simulink model "data"  (R2022a)
settings: Solver=ode1  StartTime=0.0  StopTime=100  FixedStep=0.001  RelTol=1e-3
libraries: roblocks x4
settings Model: Creator=DELL  LastModifiedBy=qinyi
settings DebuggingCC: UnconnectedInputMsg=warning  UnconnectedOutputMsg=warning  UnconnectedLineMsg=warning
settings RTWCC: DLArmComputeVersion=19.05

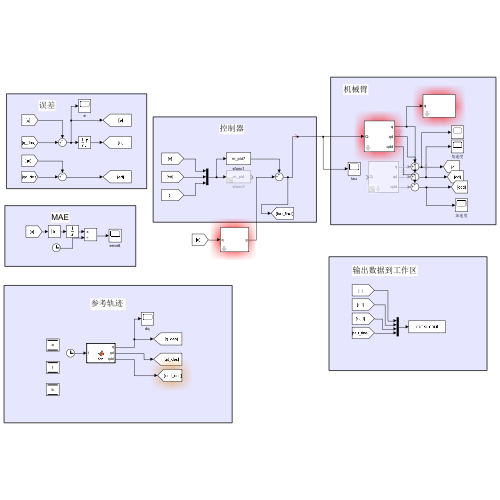
[thumbnail: Simulink's stored preview of the top-level diagram]
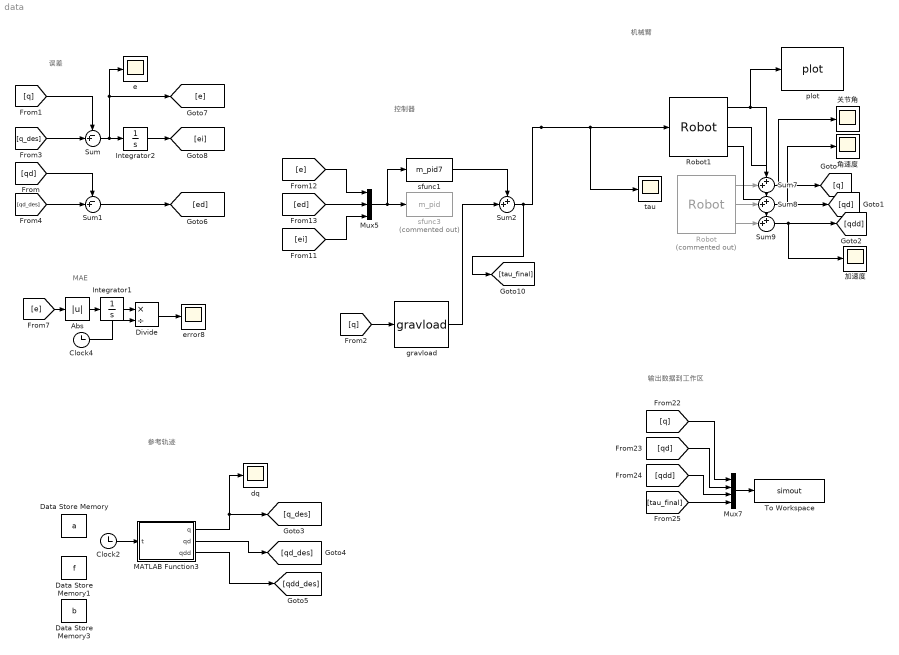
== system data ==
  note: MAE
  note: 机械臂
  note: 控制器
  note: 误差
  note: 参考轨迹
  note: 输出数据到工作区
  Abs : Abs  SaturateOnIntegerOverflow=off
  Clock2 : Clock
  Clock4 : Clock
  Data Store Memory : DataStoreMemory  DataStoreName=a  ReadBeforeWriteMsg=warning  WriteAfterWriteMsg=warning  WriteAfterReadMsg=warning  InitialValue=rand(10,7)  ShowAdditionalParam=off  OutDataTypeStr=double
  Data Store Memory1 : DataStoreMemory  DataStoreName=f  ReadBeforeWriteMsg=warning  WriteAfterWriteMsg=warning  WriteAfterReadMsg=warning  InitialValue=rand(10,7)  ShowAdditionalParam=off  OutDataTypeStr=double
  Data Store Memory3 : DataStoreMemory  DataStoreName=b  ReadBeforeWriteMsg=warning  WriteAfterWriteMsg=warning  WriteAfterReadMsg=warning  InitialValue=rand(10,7)  ShowAdditionalParam=off  OutDataTypeStr=double
  Divide : Product  Inputs=*/
  Integrator1 : Integrator
  Integrator2 : Integrator  LimitOutput=on  UpperSaturationLimit=0.01  LowerSaturationLimit=-0.01
  MATLAB Function3 : MATLAB Function  TreatAsAtomicUnit=on
  Mux5 : Mux  Inputs=3
  Mux7 : Mux
  Robot : roblocks/Arm/Robot  Commented=on  robot=p560  q0=[0 90 -90 30 0 0]*pi/180
      link override Integrator: InitialCondition=0
      link override Integrator1: InitialCondition=[0 90 -90 30 0 0]'*pi/180
      link override S-Function: Parameters=panda
  Robot1 : roblocks/Arm/Robot  robot=panda  q0=[0 90 -90 30 0 0 0]*pi/180
      link override Integrator: InitialCondition=0
      link override Integrator1: InitialCondition=[0 90 -90 30 0 0 0]'*pi/180
      link override S-Function: Parameters=panda
  Sum : Sum  Inputs=-+|
  Sum1 : Sum  Inputs=-+|
  Sum{2,7..9} (4 alike) : Sum  Inputs=++|
  To Workspace : ToWorkspace  VariableName=simout  SaveFormat=Timeseries  SampleTime=-1
  dq : Scope
  e : Scope
  error8 : Scope
  gravload : roblocks/Arm/gravload  robot=panda
  plot : roblocks/Arm/plot  robot=panda  fps=100  holdplot=on
  sfunc1 : S-Function  FunctionName=m_pid7  SFunctionDeploymentMode=off  EnableBusSupport=off
  sfunc3 : S-Function  Commented=on  FunctionName=m_pid  SFunctionDeploymentMode=off  EnableBusSupport=off
  tau : Scope
  关节角 : Scope
  加速度 : Scope
  角速度 : Scope
  wires:
  Sum/1 -> Integrator2/1, e/1, [e]
  Sum1/1 -> [ed]
  Abs/1 -> Integrator1/1
  Integrator1/1 -> Divide/1
  Divide/1 -> error8/1
  Mux5/1 -> sfunc1/1, sfunc3/1
  Mux7/1 -> To Workspace/1
  Sum7/1 -> [q], 关节角/1
  Sum8/1 -> [qd], 角速度/1
  Sum9/1 -> [qdd], 加速度/1
  Integrator2/1 -> [ei]
  Clock2/1 -> MATLAB Function3/1(t)
  MATLAB Function3/1(q) -> dq/1, [q_des]
  MATLAB Function3/2(qd) -> [qd_des]
  MATLAB Function3/3(qdd) -> [qdd_des]
  Clock4/1 -> Divide/2
  [q] -> Sum/1
  [qd] -> Sum1/1
  [q_des] -> Sum/2
  [qd_des] -> Sum1/2
  [e] -> Abs/1
  [e] -> Mux5/1
  [ed] -> Mux5/2
  [ei] -> Mux5/3
  Robot/1 -> Sum7/2
  Robot/2 -> Sum8/2
  Robot/3 -> Sum9/2
  [q] -> Mux7/1
  [qd] -> Mux7/2
  [qdd] -> Mux7/3
  [tau_final] -> Mux7/4
  sfunc1/1 -> Sum2/1
  Robot1/1 -> plot/1, Sum7/1
  Robot1/2 -> Sum8/1
  Robot1/3 -> Sum9/1
  [q] -> gravload/1
  gravload/1 -> Sum2/2
  Sum2/1 -> [tau_final], tau/1, Robot1/1

== matlab function data/MATLAB Function3 ==
  settings: updateMethod=DISCRETE
  data: t input; q output; qd output; qdd output; a data_store_memory; f data_store_memory; b data_store_memory
function [q,qd,qdd] = fcn(t)
global a;global f;global b;
if mod(t,10)==0 
    rng('shuffle');
    a=randn(10,7)-0.5;
    f=randn(10,7)*1*pi+0.2*pi;

end

B=[160 135 135 140 100 266 100]*pi/180;


q0=[B.*sum(a.*sin(b))/5]';
q=[B.*sum(a.*sin(f*t+b))/5]'+[0 90 -90 30 0 0 0]'*pi/180;
qd=[B.*sum(a.*f.*cos(f*t+b))/5]';
qdd=[B.*sum(-a.*f.*f.*sin(f*t+b))/5]';

% fq=1*ones(1,6);
% B=[80 70 70 70 50 120]*pi/180;
% q=[B.*sin(fq*t)]'+[0 90 -90 30 0 0]'*pi/180;
% qd=[B.*fq.*cos(fq*t)]';
% qdd=[-B.*fq.*fq.*sin(fq*t)]';
